simulink model "lane_stop"  (R2016a)
settings: Solver=FixedStepDiscrete  StartTime=0.0  StopTime=inf  FixedStep=0.1  RelTol=1e-3
libraries: robotlib x6
settings Model: Creator=tkikawad  LastModifiedBy=tkikawad
settings DebuggingCC: SFUnexpectedBacktrackingDiag=error  SFNoUnconditionalDefaultTransitionDiag=error
settings GRTTargetCC: TargetLangStandard=C99 (ISO)  GeneratePreprocessorConditionals=Use local settings
settings ConfigComp: CovMetricSettings=dwe  CovHtmlReporting=off  CovSaveCumulativeToWorkspaceVar=off  CovSaveSingleToWorkspaceVar=off  CovExternalEMLEnable=on

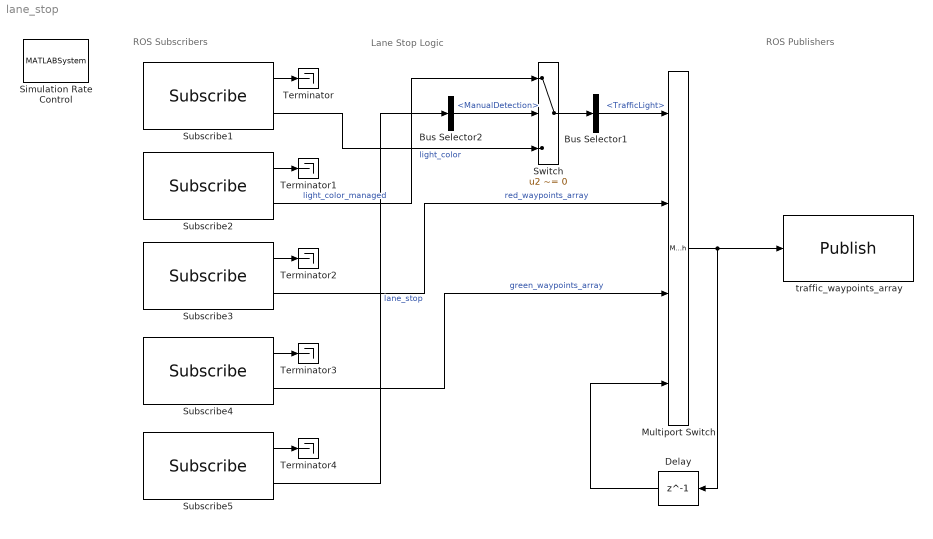
== system lane_stop ==
  note: Lane Stop Logic
  note: ROS Publishers
  note: ROS Subscribers
  Bus Selector1 : BusSelector  OutputSignals=TrafficLight
  Bus Selector2 : BusSelector  OutputSignals=ManualDetection
  Delay : Delay  DelayLength=1
  Multiport Switch : MultiPortSwitch  DiagnosticForDefault=None
  Simulation Rate Control : MATLABSystem  System=ExampleHelperSimulationRateControl  SampleTime=0.1
      mask Type: ExampleHelperSimulationRateControl
      mask Display: disp('Rate Control');
  Subscribe1 : robotlib/Subscribe  SourceLibraryInfo=This block requires Robotics System Toolbox  topicSource=Specify your own  topic=/light_color  messageType=autoware_msgs/traffic_light  sampleTime=-1  messageQueueLength=1
  Subscribe2 : robotlib/Subscribe  SourceLibraryInfo=This block requires Robotics System Toolbox  topicSource=Specify your own  topic=/light_color_managed  messageType=autoware_msgs/traffic_light  sampleTime=-1  messageQueueLength=1
  Subscribe3 : robotlib/Subscribe  SourceLibraryInfo=This block requires Robotics System Toolbox  topicSource=Specify your own  topic=/red_waypoints_array  messageType=autoware_msgs/LaneArray  sampleTime=-1  messageQueueLength=1
  Subscribe4 : robotlib/Subscribe  SourceLibraryInfo=This block requires Robotics System Toolbox  topicSource=Specify your own  topic=/green_waypoints_array  messageType=autoware_msgs/LaneArray  sampleTime=-1  messageQueueLength=1
  Subscribe5 : robotlib/Subscribe  SourceLibraryInfo=This block requires Robotics System Toolbox  topicSource=Specify your own  topic=/config/lane_stop  messageType=autoware_msgs/ConfigLaneStop  sampleTime=-1  messageQueueLength=1
  Switch : Switch  Criteria=u2 ~= 0  Threshold=t  ZeroCross=off
  Terminator{,1..4} (5 alike) : Terminator
  traffic_waypoints_array : robotlib/Publish  SourceLibraryInfo=This block requires Robotics System Toolbox  topicSource=Specify your own  topic=/traffic_waypoints_array  messageType=autoware_msgs/LaneArray  messageQueueLength=1
  wires:
  Bus Selector2/1 -> Switch/2  "<ManualDetection>"
  Switch/1 -> Bus Selector1/1
  Bus Selector1/1 -> Multiport Switch/1  "<TrafficLight>"
  Subscribe1/1 -> Terminator/1
  Subscribe3/1 -> Terminator2/1
  Subscribe5/1 -> Terminator4/1
  Subscribe2/1 -> Terminator1/1
  Subscribe4/1 -> Terminator3/1
  Subscribe5/2 -> Bus Selector2/1  "lane_stop"
  Subscribe4/2 -> Multiport Switch/3  "green_waypoints_array"
  Subscribe1/2 -> Switch/3  "light_color"
  Subscribe3/2 -> Multiport Switch/2  "red_waypoints_array"
  Subscribe2/2 -> Switch/1  "light_color_managed"
  Delay/1 -> Multiport Switch/4
  Multiport Switch/1 -> traffic_waypoints_array/1, Delay/1
